simulink model "Case2_ASMC"  (R2019a)
settings: Solver=ode4  StartTime=0.0  StopTime=t(end)  FixedStep=dt  RelTol=1e-3
values from neighbouring files (symbols this model uses):
  coe = [c1 c2 c3]    [Case2.m]
  dt = 1/4096    (= 0.000244140625)    [Case2.m]
  k0 = 20    [Case2.m]
  Para = [alpha_hat0 b_hat0 alpha_bar b_bar lambda lambda1 eta sw]    [Case2.m]
  Psi_hat0 = [alpha_hat0;b_hat0]    [Case2.m]
  theta0 = 10    [Case2.m]
  x1d = zeros(Nt,1)    [Case2.m]
settings Model: Creator=hongwei  LastModifiedBy=hongwei
settings DataIOCC: SaveTime=off  ReturnWorkspaceOutputs=off

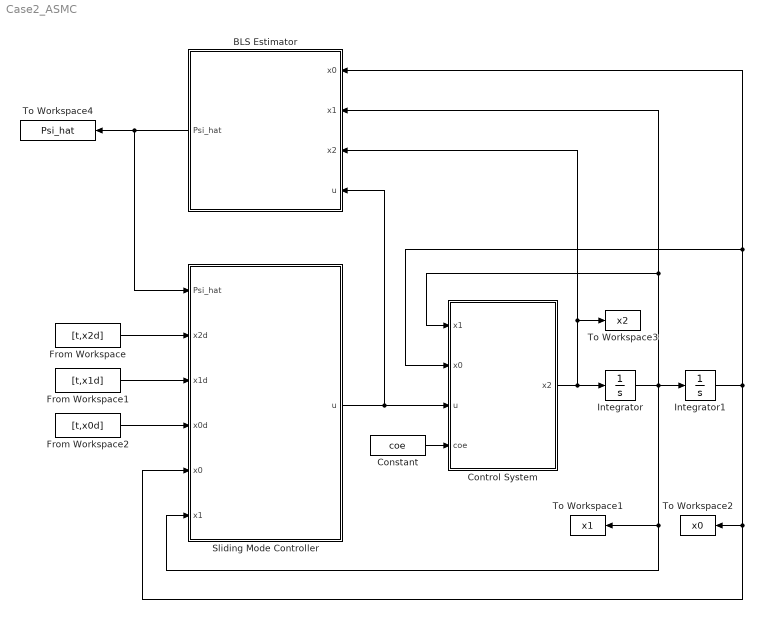
== system Case2_ASMC ==
  BLS Estimator : Subsystem
  Constant : Constant  Value=coe  VectorParams1D=off
  Control System : MATLAB Function  TreatAsAtomicUnit=on
  From Workspace : FromWorkspace  VariableName=[t,x2d]  SampleTime=dt
  From Workspace1 : FromWorkspace  VariableName=[t,x1d]  SampleTime=dt
  From Workspace2 : FromWorkspace  VariableName=[t,x0d]  SampleTime=dt
  Integrator : Integrator  InitialCondition=x1d(1)
  Integrator1 : Integrator
  Sliding Mode Controller : Subsystem
  To Workspace1 : ToWorkspace  VariableName=x1  SampleTime=-1
  To Workspace2 : ToWorkspace  VariableName=x0  SampleTime=-1
  To Workspace3 : ToWorkspace  VariableName=x2  SampleTime=-1
  To Workspace4 : ToWorkspace  VariableName=Psi_hat  SampleTime=-1
  wires:
  From Workspace/1 -> Sliding Mode Controller/2(x2d)
  From Workspace1/1 -> Sliding Mode Controller/3(x1d)
  From Workspace2/1 -> Sliding Mode Controller/4(x0d)
  Control System/1(x2) -> BLS Estimator/3(x2), To Workspace3/1, Integrator/1
  Integrator/1 -> BLS Estimator/2(x1), Control System/1(x1), Integrator1/1, To Workspace1/1, Sliding Mode Controller/6(x1)
  Integrator1/1 -> BLS Estimator/1(x0), Control System/2(x0), Sliding Mode Controller/5(x0), To Workspace2/1
  Constant/1 -> Control System/4(coe)
  Sliding Mode Controller/1(u) -> BLS Estimator/4(u), Control System/3(u)
  BLS Estimator/1(Psi_hat) -> To Workspace4/1, Sliding Mode Controller/1(Psi_hat)

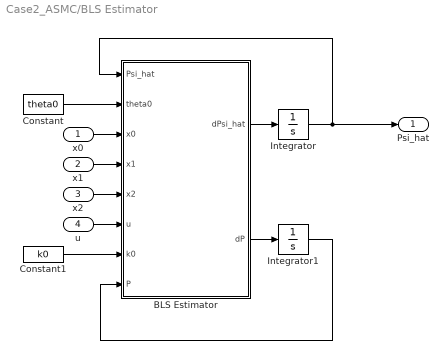
== system Case2_ASMC/BLS Estimator ==
  x0 : Inport
  x1 : Inport  Port=2
  x2 : Inport  Port=3
  u : Inport  Port=4
  BLS Estimator : MATLAB Function  TreatAsAtomicUnit=on
  Constant : Constant  Value=theta0
  Constant1 : Constant  Value=k0
  Integrator : Integrator  InitialCondition=Psi_hat0
  Integrator1 : Integrator  InitialCondition=k0*eye(2)
  Psi_hat : Outport
  wires:
  x0/1 -> BLS Estimator/3(x0)
  x1/1 -> BLS Estimator/4(x1)
  x2/1 -> BLS Estimator/5(x2)
  u/1 -> BLS Estimator/6(u)
  BLS Estimator/1(dPsi_hat) -> Integrator/1
  Integrator/1 -> Psi_hat/1, BLS Estimator/1(Psi_hat)
  BLS Estimator/2(dP) -> Integrator1/1
  Integrator1/1 -> BLS Estimator/8(P)
  Constant/1 -> BLS Estimator/2(theta0)
  Constant1/1 -> BLS Estimator/7(k0)

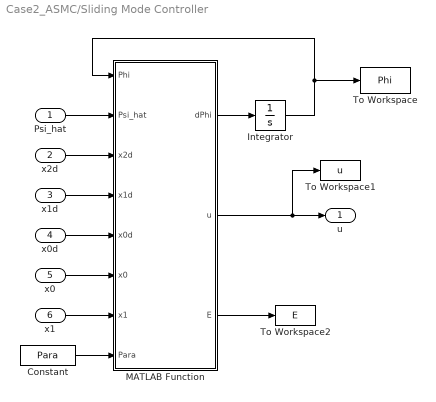
== system Case2_ASMC/Sliding Mode Controller ==
  Psi_hat : Inport
  x2d : Inport  Port=2
  x1d : Inport  Port=3
  x0d : Inport  Port=4
  x0 : Inport  Port=5
  x1 : Inport  Port=6
  Constant : Constant  Value=Para  VectorParams1D=off
  Integrator : Integrator
  MATLAB Function : MATLAB Function  TreatAsAtomicUnit=on
  To Workspace : ToWorkspace  VariableName=Phi  SampleTime=-1
  To Workspace1 : ToWorkspace  VariableName=u  SampleTime=-1
  To Workspace2 : ToWorkspace  VariableName=E  SampleTime=-1
  u : Outport
  wires:
  Constant/1 -> MATLAB Function/8(Para)
  x1d/1 -> MATLAB Function/4(x1d)
  MATLAB Function/2(u) -> u/1, To Workspace1/1
  MATLAB Function/1(dPhi) -> Integrator/1
  Integrator/1 -> To Workspace/1, MATLAB Function/1(Phi)
  x2d/1 -> MATLAB Function/3(x2d)
  x0d/1 -> MATLAB Function/5(x0d)
  x0/1 -> MATLAB Function/6(x0)
  x1/1 -> MATLAB Function/7(x1)
  MATLAB Function/3(E) -> To Workspace2/1
  Psi_hat/1 -> MATLAB Function/2(Psi_hat)

== matlab function Case2_ASMC/Control System ==
  data: x1 input; x0 input; u input; coe input; x2 output
function x2 = SYS(x1,x0,u,coe)
c1=coe(1); c2=coe(2); c3=coe(3);
x2=-c1*x0-c2*(x0^2-1)*x1+c3*u;

== matlab function Case2_ASMC/Sliding Mode Controller/MATLAB Function ==
  data: Phi input; Psi_hat input; x2d input; x1d input; dPhi output; x0d input; x0 input; x1 input; Para input; u output; E output
function [dPhi,u,E] = SMC(Phi,Psi_hat,x2d,x1d,x0d,x0,x1,Para)
alpha_hat=Psi_hat(1)';
b_hat=Psi_hat(2);
a_bar=Para(3);
b_bar=Para(4);
lambda=Para(5);
lambda1=Para(6);
eta=Para(7);
sw=Para(8);

% f=x1^2*cos(3*x0);
f=x0;
e0=x0-x0d; e1=x1-x1d;
E=e1+lambda*e0;
h=x2d-lambda*e1;
bu_hat=alpha_hat*f+h;
u_hat=bu_hat/b_hat;

rho1=b_hat/(b_hat-sign(b_hat)*b_bar);
k0=rho1*a_bar*abs(f)+(rho1-1)*abs(bu_hat);

if sw~=0
    rho2=b_hat/(b_hat+sign(b_hat)*b_bar);
    k=lambda1*rho2*Phi;
    k_=k-k0;
    if k_<0
        dPhi=eta-k_/rho2;
    else
        dPhi=eta-k_/rho1;
    end
else
    k=k0+rho1*eta;
    dPhi=0;
end
if abs(E)>=Phi
    sat=sign(E);
else
    sat=E/Phi;
end
uc=-k*sat/b_hat;
u=u_hat+uc;

== matlab function Case2_ASMC/BLS Estimator/BLS Estimator ==
  data: Psi_hat input; theta0 input; x0 input; x1 input; x2 input; u input; k0 input; P input; dPsi_hat output; dP output
function [dPsi_hat,dP] = BLS(Psi_hat,theta0,x0,x1,x2,u,k0,P)
y=x2;
% W=[-x1^2*cos(3*x0) u];
W=[-x0 u];
yhat=W*Psi_hat;
e1=yhat-y;
dPsi_hat=-P*W'*e1;
theta=theta0*(1-norm(P)/k0);
dP=theta*P-P*(W'*W)*P;
